simulink library "Pitch_System_Lib"  (Simulink 7.9)
settings: Solver=ode45  StartTime=0.0  StopTime=10.0  RelTol=1e-3
undefined symbols (not defined in the file or in its folder): WT_Params
libraries: mblibv1 x78, Pitch_Actuation_Lib x2, Pitch_System_Lib x1
(part 2 of 5)

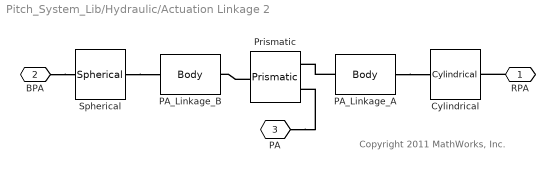
== system Pitch_System_Lib/Hydraulic/Actuation Linkage 2 ==
  note: Copyright 2011 MathWorks, Inc.
  Cylindrical : mblibv1/Joints/Cylindrical  PhysicalDomain=mechanical  SubClassName=Unknown  LeftPortType=blob  RightPortType=blob  LConnTagsString=__newl0  RConnTagsString=__newr0  UpdateFromCAD=off  NumSAPorts=0  CutJoint=off  MarkAsCut=off  Primitives=prismatic  PrimitiveProps=P1$Follower$[0 1 0]$prismatic#R1$Follower$[0 1 0]$revolute  DialogClass=JointBlock  P1Axis=[0 1 0]  R1Axis=[0 1 0]
  PA_Linkage_A : mblibv1/Bodies/Body  PhysicalDomain=mechanical  SubClassName=Unknown  LeftPortType=workingframe  RightPortType=workingframe  LConnTagsString=CS2  RConnTagsString=CS1  UpdateFromCAD=off  DialogClass=MechanicalBodyBlock  Mass=WT_Params.Pitch_Actuator.cylinder_mass  MassUnits=kg  InertiaUnits=kg*m^2  Inertia=WT_Params.Pitch_Actuator.cylinder_inertia  Shape=Cylinder  ShapeDims=[1 1]  ShapeUnits=m  ShapeUse=false  Density=1  DensityUnits=kg/m^3  DensityUse=false  GraphicsMode=MACHINE_DEFAULT  BodyColorSelMode=COLORPALETTE  BodyColor="[1     0.56863    0.011765]"  AttachedToCS=CG  CG=Left$CG$[WT_Params.Pitch_Actuator.cylinder_length/2 0 0]$CS2$CS2$m$[0 0 0]$Euler X-Y-Z$deg$CS1$false$none  WorkingFrames="Right$CS1$[WT_Params.Pitch_Actuator.cylinder_length 0 0]$CS2$CS2$m$[0 0 0]$Euler X-Y-Z$deg$Adjoining$true$none#Left$CS2$[0 0 0]$Adjoining$Adjoining$m$[0 0 0]$Euler X-Y-Z$deg$CS1$true$none#Right$CS7$[0 WT_Params.Pitch_Actuator.Geometry.outer_radius*cos(0)  WT_Params.Pitch_Actuator.Geometry.outer_radius*sin(0)]$CS1$CS1$m$[0 0 0]$Euler X-Y-Z$deg$CS1$false$none#Right$CS8$[0 WT_Params.Pitch_Actuator.Geometry.outer_radius*cos(0.2*pi)  WT_Params.Pitch_Actuator.Geometry.outer_radius*sin(0.2*pi)]$CS1$CS1$m$[0 0 0]$Euler X-Y-Z$deg$CS1$false$none#Right$CS9$[0 WT_Params.Pitch_Actuator.Geometry.outer_radius*cos(0.4*pi)  WT_Params.Pitch_Actuator.Geometry.outer_radius*sin(0.4*pi)]$CS1$CS1$m$[0 0 0]$Euler X-Y-Z$deg$CS1$false$none#Right$CS10$[0 WT_Params.Pitch_Actuator.Geometry.outer_radius*cos(0.6*pi)  WT_Params.Pitch_Actuator.Geometry.outer_radius*sin(0.6*pi)]$CS1$CS1$m$[0 0 0]$Euler X-Y-Z$deg$CS1$false$none#Right$CS11$[0 WT_Params.Pitch_Actuator.Geometry.outer_radius*cos(0.8*pi)  WT_Params.Pitch_Actuator.Geometry.outer_radius*sin(0.8*pi)]$CS1$CS1$m$[0 0 0]$Euler X-Y-Z$deg$CS1$false$none#Right$CS12$[0 WT_Params.Pitch_Actuator.Geometry.outer_radius*cos(1.0*pi)  WT_Params.Pitch_Actuator.Geometry.outer_radius*sin(1.0*pi)]$CS1$CS1$m$[0 0 0]$Euler X-Y-Z$deg$CS1$false$none#Right$CS13$[0 WT_Params.Pitch_Actuator.Geometry.outer_radius*cos(1.2*pi)  WT_Params.Pitch_Actuator.Geometry.outer_radius*sin(1.2*pi)]$CS1$CS1$m$[0 0 0]$Euler X-Y-Z$deg$CS1$false$none#Right$CS14$[0 WT_Params.Pitch_Actuator.Geometry.outer_radius*cos(1.4*pi)  WT_Params.Pitch_Actuator.Geometry.outer_radius*sin(1.4*pi)]$CS1$CS1$m$[0 0 0]$Euler X-Y-Z$deg$CS1$false$none#Right$CS15$[0 WT_Params.Pitch_Actuator.Geometry.outer_radius*cos(1.6*pi)  WT_Params.Pitch_Actuator.Geometry.outer_radius*sin(1.6*pi)]$CS1$CS1$m$[0 0 0]$Euler X-Y-Z$deg$CS1$false$none#Right$CS16$[0 WT_Params.Pitch_Actuator.Geometry.outer_radius*cos(1.8*pi)  WT_Params.Pitch_Actuator.Geometry.outer_radius*sin(1.8*pi)]$CS1$CS1$m$[0 0 0]$Euler X-Y-Z$deg$CS1$false$none#Right$CS17$[-WT_Params.Pitch_Actuator.cylinder_length WT_Params.Pitch_Actuator.Geometry.outer_radius*cos(0)  WT_Params.Pitch_Actuator.Geometry.outer_radius*sin(0)]$CS1$CS1$m$[0 0 0]$Euler X-Y-Z$deg$CS1$false$none#Right$CS18$[-WT_Params.Pitch_Actuator.cylinder_length WT_Params.Pitch_Actuator.Geometry.outer_radius*cos(0.2*pi)  WT_Params.Pitch_Actuator.Geometry.outer_radius*sin(0.2*pi)]$CS1$CS1$m$[0 0 0]$Euler X-Y-Z$deg$CS1$false$none#Right$CS19$[-WT_Params.Pitch_Actuator.cylinder_length WT_Params.Pitch_Actuator.Geometry.outer_radius*cos(0.4*pi)  WT_Params.Pitch_Actuator.Geometry.outer_radius*sin(0.4*pi)]$CS1$CS1$m$[0 0 0]$Euler X-Y-Z$deg$CS1$false$none#Right$CS20$[-WT_Params.Pitch_Actuator.cylinder_length WT_Params.Pitch_Actuator.Geometry.outer_radius*cos(0.6*pi)  WT_Params.Pitch_Actuator.Geometry.outer_radius*sin(0.6*pi)]$CS1$CS1$m$[0 0 0]$Euler X-Y-Z$deg$CS1$false$none#Right$CS21$[-WT_Params.Pitch_Actuator.cylinder_length WT_Params.Pitch_Actuator.Geometry.outer_radius*cos(0.8*pi)  WT_Params.Pitch_Actuator.Geometry.outer_radius*sin(0.8*pi)]$CS1$CS1$m$[0 0 0]$Euler X-Y-Z$deg$CS1$false$none#Right$CS22$[-WT_Params.Pitch_Actuator.cylinder_length WT_Params.Pitch_Actuator.Geometry.outer_radius*cos(1.0*pi)  WT_Params.Pitch_Actuator.Geometry.outer_radius*sin(1.0*pi)]$CS1$CS1$m$[0 0 0]$Euler X-Y-Z$deg$CS1$false$none#Right$CS23$[-WT_Params.Pitch_Actuator.cylinder_length WT_Params.Pitch_Actuator.Geometry.outer_radius*cos(1.2*pi)  WT_Params.Pitch_Actuator.Geometry.outer_radius*sin(1.2*pi)]$CS1$CS1$m$[0 0 0]$Euler X-Y-Z$deg$CS1$false$none#Right$CS24$[-WT_Params.Pitch_Actuator.cylinder_length WT_Params.Pitch_Actuator.Geometry.outer_radius*cos(1.4*pi)  WT_Params.Pitch_Actuator.Geometry.outer_radius*sin(1.4*pi)]$CS1$CS1$m$[0 0 0]$Euler X-Y-Z$deg$CS1$false$none#Right$CS25$[-WT_Params.Pitch_Actuator.cylinder_length WT_Params.Pitch_Actuator.Geometry.outer_radius*cos(1.6*pi)  WT_Params.Pitch_Actuator.Geometry.outer_radius*sin(1.6*pi)]$CS1$CS1$m$[0 0 0]$Euler X-Y-Z$deg$CS1$false$none#Right$CS26$[-WT_Params.Pitch_Actuator.cylinder_length WT_Params.Pitch_Actuator.Geometry.outer_radius*cos(1.8*pi)  WT_Params.Pitch_Actuator.Geometry.outer_radius*sin(1.8*pi)]$CS1$CS1$m$[0 0 0]$Euler X-Y-Z$deg$CS1$false$none"  CGPos=[WT_Params.Pitch_Actuator.cylinder_length/2 0 0]  CGRot=[0 0 0]  CS0Pos=[]  CS0Rot=[]  CS1Pos=[WT_Params.Pitch_Actuator.cylinder_length 0 0]  CS1Rot=[0 0 0]  CS2Pos=[0 0 0]  CS2Rot=[0 0 0]  CS3Pos=[]  CS3Rot=[]  CS4Pos=[]  CS4Rot=[]  CS5Pos=[]  CS5Rot=[]  CS6Pos=[]  CS6Rot=[]  CS7Pos="[0 WT_Params.Pitch_Actuator.Geometry.outer_radius*cos(0)  WT_Params.Pitch_Actuator.Geometry.outer_radius*sin(0)]"  CS7Rot=[0 0 0]  CS8Pos="[0 WT_Params.Pitch_Actuator.Geometry.outer_radius*cos(0.2*pi)  WT_Params.Pitch_Actuator.Geometry.outer_radius*sin(0.2*pi)]"  CS8Rot=[0 0 0]  CS9Pos="[0 WT_Params.Pitch_Actuator.Geometry.outer_radius*cos(0.4*pi)  WT_Params.Pitch_Actuator.Geometry.outer_radius*sin(0.4*pi)]"  CS9Rot=[0 0 0]  CS10Pos="[0 WT_Params.Pitch_Actuator.Geometry.outer_radius*cos(0.6*pi)  WT_Params.Pitch_Actuator.Geometry.outer_radius*sin(0.6*pi)]"  CS10Rot=[0 0 0]  CS11Pos="[0 WT_Params.Pitch_Actuator.Geometry.outer_radius*cos(0.8*pi)  WT_Params.Pitch_Actuator.Geometry.outer_radius*sin(0.8*pi)]"  CS11Rot=[0 0 0]  CS12Pos="[0 WT_Params.Pitch_Actuator.Geometry.outer_radius*cos(1.0*pi)  WT_Params.Pitch_Actuator.Geometry.outer_radius*sin(1.0*pi)]"  CS12Rot=[0 0 0]  CS13Pos="[0 WT_Params.Pitch_Actuator.Geometry.outer_radius*cos(1.2*pi)  WT_Params.Pitch_Actuator.Geometry.outer_radius*sin(1.2*pi)]"  CS13Rot=[0 0 0]  CS14Pos="[0 WT_Params.Pitch_Actuator.Geometry.outer_radius*cos(1.4*pi)  WT_Params.Pitch_Actuator.Geometry.outer_radius*sin(1.4*pi)]"  CS14Rot=[0 0 0]  CS15Pos="[0 WT_Params.Pitch_Actuator.Geometry.outer_radius*cos(1.6*pi)  WT_Params.Pitch_Actuator.Geometry.outer_radius*sin(1.6*pi)]"  CS15Rot=[0 0 0]  CS16Pos="[0 WT_Params.Pitch_Actuator.Geometry.outer_radius*cos(1.8*pi)  WT_Params.Pitch_Actuator.Geometry.outer_radius*sin(1.8*pi)]"  CS16Rot=[0 0 0]  CS17Pos="[-WT_Params.Pitch_Actuator.cylinder_length WT_Params.Pitch_Actuator.Geometry.outer_radius*cos(0)  WT_Params.Pitch_Actuator.Geometry.outer_radius*sin(0)]"  CS17Rot=[0 0 0]  CS18Pos="[-WT_Params.Pitch_Actuator.cylinder_length WT_Params.Pitch_Actuator.Geometry.outer_radius*cos(0.2*pi)  WT_Params.Pitch_Actuator.Geometry.outer_radius*sin(0.2*pi)]"  CS18Rot=[0 0 0]  CS19Pos="[-WT_Params.Pitch_Actuator.cylinder_length WT_Params.Pitch_Actuator.Geometry.outer_radius*cos(0.4*pi)  WT_Params.Pitch_Actuator.Geometry.outer_radius*sin(0.4*pi)]"  CS19Rot=[0 0 0]  CS20Pos="[-WT_Params.Pitch_Actuator.cylinder_length WT_Params.Pitch_Actuator.Geometry.outer_radius*cos(0.6*pi)  WT_Params.Pitch_Actuator.Geometry.outer_radius*sin(0.6*pi)]"  CS20Rot=[0 0 0]
  PA_Linkage_B : mblibv1/Bodies/Body  PhysicalDomain=mechanical  SubClassName=Unknown  LeftPortType=workingframe  RightPortType=workingframe  LConnTagsString=CS2  RConnTagsString=CS1  UpdateFromCAD=off  DialogClass=MechanicalBodyBlock  Mass=WT_Params.Pitch_Actuator.rod_mass  MassUnits=kg  InertiaUnits=kg*m^2  Inertia=WT_Params.Pitch_Actuator.rod_inertia  Shape=Cylinder  ShapeDims=[1 1]  ShapeUnits=m  ShapeUse=false  Density=1  DensityUnits=kg/m^3  DensityUse=false  GraphicsMode=MACHINE_DEFAULT  BodyColorSelMode=COLORPALETTE  BodyColor="[0.31373     0.31765     0.31373]"  AttachedToCS=CG  CG=Left$CG$[-WT_Params.Pitch_Actuator.cylinder_length/2 0 0]$CS1$CS1$m$[0 0 0]$Euler X-Y-Z$deg$CS1$false$none  WorkingFrames="Right$CS1$[0 0 0]$Adjoining$Adjoining$m$[0 0 0]$Euler X-Y-Z$deg$Adjoining$true$none#Left$CS2$[-WT_Params.Pitch_Actuator.cylinder_length 0 0]$CS1$CS1$m$[0 0 0]$Euler X-Y-Z$deg$CS1$true$none#Right$CS7$[0 WT_Params.Pitch_Actuator.Geometry.inner_radius*cos(0)  WT_Params.Pitch_Actuator.Geometry.inner_radius*sin(0)]$CS1$CS1$m$[0 0 0]$Euler X-Y-Z$deg$CS1$false$none#Right$CS8$[0 WT_Params.Pitch_Actuator.Geometry.inner_radius*cos(0.2*pi)  WT_Params.Pitch_Actuator.Geometry.inner_radius*sin(0.2*pi)]$CS1$CS1$m$[0 0 0]$Euler X-Y-Z$deg$CS1$false$none#Right$CS9$[0 WT_Params.Pitch_Actuator.Geometry.inner_radius*cos(0.4*pi)  WT_Params.Pitch_Actuator.Geometry.inner_radius*sin(0.4*pi)]$CS1$CS1$m$[0 0 0]$Euler X-Y-Z$deg$CS1$false$none#Right$CS10$[0 WT_Params.Pitch_Actuator.Geometry.inner_radius*cos(0.6*pi)  WT_Params.Pitch_Actuator.Geometry.inner_radius*sin(0.6*pi)]$CS1$CS1$m$[0 0 0]$Euler X-Y-Z$deg$CS1$false$none#Right$CS11$[0 WT_Params.Pitch_Actuator.Geometry.inner_radius*cos(0.8*pi)  WT_Params.Pitch_Actuator.Geometry.inner_radius*sin(0.8*pi)]$CS1$CS1$m$[0 0 0]$Euler X-Y-Z$deg$CS1$false$none#Right$CS12$[0 WT_Params.Pitch_Actuator.Geometry.inner_radius*cos(1.0*pi)  WT_Params.Pitch_Actuator.Geometry.inner_radius*sin(1.0*pi)]$CS1$CS1$m$[0 0 0]$Euler X-Y-Z$deg$CS1$false$none#Right$CS13$[0 WT_Params.Pitch_Actuator.Geometry.inner_radius*cos(1.2*pi)  WT_Params.Pitch_Actuator.Geometry.inner_radius*sin(1.2*pi)]$CS1$CS1$m$[0 0 0]$Euler X-Y-Z$deg$CS1$false$none#Right$CS14$[0 WT_Params.Pitch_Actuator.Geometry.inner_radius*cos(1.4*pi)  WT_Params.Pitch_Actuator.Geometry.inner_radius*sin(1.4*pi)]$CS1$CS1$m$[0 0 0]$Euler X-Y-Z$deg$CS1$false$none#Right$CS15$[0 WT_Params.Pitch_Actuator.Geometry.inner_radius*cos(1.6*pi)  WT_Params.Pitch_Actuator.Geometry.inner_radius*sin(1.6*pi)]$CS1$CS1$m$[0 0 0]$Euler X-Y-Z$deg$CS1$false$none#Right$CS16$[0 WT_Params.Pitch_Actuator.Geometry.inner_radius*cos(1.8*pi)  WT_Params.Pitch_Actuator.Geometry.inner_radius*sin(1.8*pi)]$CS1$CS1$m$[0 0 0]$Euler X-Y-Z$deg$CS1$false$none#Right$CS17$[-WT_Params.Pitch_Actuator.cylinder_length WT_Params.Pitch_Actuator.Geometry.inner_radius*cos(0)  WT_Params.Pitch_Actuator.Geometry.inner_radius*sin(0)]$CS1$CS1$m$[0 0 0]$Euler X-Y-Z$deg$CS1$false$none#Right$CS18$[-WT_Params.Pitch_Actuator.cylinder_length WT_Params.Pitch_Actuator.Geometry.inner_radius*cos(0.2*pi)  WT_Params.Pitch_Actuator.Geometry.inner_radius*sin(0.2*pi)]$CS1$CS1$m$[0 0 0]$Euler X-Y-Z$deg$CS1$false$none#Right$CS19$[-WT_Params.Pitch_Actuator.cylinder_length WT_Params.Pitch_Actuator.Geometry.inner_radius*cos(0.4*pi)  WT_Params.Pitch_Actuator.Geometry.inner_radius*sin(0.4*pi)]$CS1$CS1$m$[0 0 0]$Euler X-Y-Z$deg$CS1$false$none#Right$CS20$[-WT_Params.Pitch_Actuator.cylinder_length WT_Params.Pitch_Actuator.Geometry.inner_radius*cos(0.6*pi)  WT_Params.Pitch_Actuator.Geometry.inner_radius*sin(0.6*pi)]$CS1$CS1$m$[0 0 0]$Euler X-Y-Z$deg$CS1$false$none#Right$CS21$[-WT_Params.Pitch_Actuator.cylinder_length WT_Params.Pitch_Actuator.Geometry.inner_radius*cos(0.8*pi)  WT_Params.Pitch_Actuator.Geometry.inner_radius*sin(0.8*pi)]$CS1$CS1$m$[0 0 0]$Euler X-Y-Z$deg$CS1$false$none#Right$CS22$[-WT_Params.Pitch_Actuator.cylinder_length WT_Params.Pitch_Actuator.Geometry.inner_radius*cos(1.0*pi)  WT_Params.Pitch_Actuator.Geometry.inner_radius*sin(1.0*pi)]$CS1$CS1$m$[0 0 0]$Euler X-Y-Z$deg$CS1$false$none#Right$CS23$[-WT_Params.Pitch_Actuator.cylinder_length WT_Params.Pitch_Actuator.Geometry.inner_radius*cos(1.2*pi)  WT_Params.Pitch_Actuator.Geometry.inner_radius*sin(1.2*pi)]$CS1$CS1$m$[0 0 0]$Euler X-Y-Z$deg$CS1$false$none#Right$CS24$[-WT_Params.Pitch_Actuator.cylinder_length WT_Params.Pitch_Actuator.Geometry.inner_radius*cos(1.4*pi)  WT_Params.Pitch_Actuator.Geometry.inner_radius*sin(1.4*pi)]$CS1$CS1$m$[0 0 0]$Euler X-Y-Z$deg$CS1$false$none#Right$CS25$[-WT_Params.Pitch_Actuator.cylinder_length WT_Params.Pitch_Actuator.Geometry.inner_radius*cos(1.6*pi)  WT_Params.Pitch_Actuator.Geometry.inner_radius*sin(1.6*pi)]$CS1$CS1$m$[0 0 0]$Euler X-Y-Z$deg$CS1$false$none#Right$CS26$[-WT_Params.Pitch_Actuator.cylinder_length WT_Params.Pitch_Actuator.Geometry.inner_radius*cos(1.8*pi)  WT_Params.Pitch_Actuator.Geometry.inner_radius*sin(1.8*pi)]$CS1$CS1$m$[0 0 0]$Euler X-Y-Z$deg$CS1$false$none"  CGPos=[-WT_Params.Pitch_Actuator.cylinder_length/2 0 0]  CGRot=[0 0 0]  CS0Pos=[]  CS0Rot=[]  CS1Pos=[0 0 0]  CS1Rot=[0 0 0]  CS2Pos=[-WT_Params.Pitch_Actuator.cylinder_length 0 0]  CS2Rot=[0 0 0]  CS3Pos=[]  CS3Rot=[]  CS4Pos=[]  CS4Rot=[]  CS5Pos=[]  CS5Rot=[]  CS6Pos=[]  CS6Rot=[]  CS7Pos="[0 WT_Params.Pitch_Actuator.Geometry.inner_radius*cos(0)  WT_Params.Pitch_Actuator.Geometry.inner_radius*sin(0)]"  CS7Rot=[0 0 0]  CS8Pos="[0 WT_Params.Pitch_Actuator.Geometry.inner_radius*cos(0.2*pi)  WT_Params.Pitch_Actuator.Geometry.inner_radius*sin(0.2*pi)]"  CS8Rot=[0 0 0]  CS9Pos="[0 WT_Params.Pitch_Actuator.Geometry.inner_radius*cos(0.4*pi)  WT_Params.Pitch_Actuator.Geometry.inner_radius*sin(0.4*pi)]"  CS9Rot=[0 0 0]  CS10Pos="[0 WT_Params.Pitch_Actuator.Geometry.inner_radius*cos(0.6*pi)  WT_Params.Pitch_Actuator.Geometry.inner_radius*sin(0.6*pi)]"  CS10Rot=[0 0 0]  CS11Pos="[0 WT_Params.Pitch_Actuator.Geometry.inner_radius*cos(0.8*pi)  WT_Params.Pitch_Actuator.Geometry.inner_radius*sin(0.8*pi)]"  CS11Rot=[0 0 0]  CS12Pos="[0 WT_Params.Pitch_Actuator.Geometry.inner_radius*cos(1.0*pi)  WT_Params.Pitch_Actuator.Geometry.inner_radius*sin(1.0*pi)]"  CS12Rot=[0 0 0]  CS13Pos="[0 WT_Params.Pitch_Actuator.Geometry.inner_radius*cos(1.2*pi)  WT_Params.Pitch_Actuator.Geometry.inner_radius*sin(1.2*pi)]"  CS13Rot=[0 0 0]  CS14Pos="[0 WT_Params.Pitch_Actuator.Geometry.inner_radius*cos(1.4*pi)  WT_Params.Pitch_Actuator.Geometry.inner_radius*sin(1.4*pi)]"  CS14Rot=[0 0 0]  CS15Pos="[0 WT_Params.Pitch_Actuator.Geometry.inner_radius*cos(1.6*pi)  WT_Params.Pitch_Actuator.Geometry.inner_radius*sin(1.6*pi)]"  CS15Rot=[0 0 0]  CS16Pos="[0 WT_Params.Pitch_Actuator.Geometry.inner_radius*cos(1.8*pi)  WT_Params.Pitch_Actuator.Geometry.inner_radius*sin(1.8*pi)]"  CS16Rot=[0 0 0]  CS17Pos="[-WT_Params.Pitch_Actuator.cylinder_length WT_Params.Pitch_Actuator.Geometry.inner_radius*cos(0)  WT_Params.Pitch_Actuator.Geometry.inner_radius*sin(0)]"  CS17Rot=[0 0 0]  CS18Pos="[-WT_Params.Pitch_Actuator.cylinder_length WT_Params.Pitch_Actuator.Geometry.inner_radius*cos(0.2*pi)  WT_Params.Pitch_Actuator.Geometry.inner_radius*sin(0.2*pi)]"  CS18Rot=[0 0 0]  CS19Pos="[-WT_Params.Pitch_Actuator.cylinder_length WT_Params.Pitch_Actuator.Geometry.inner_radius*cos(0.4*pi)  WT_Params.Pitch_Actuator.Geometry.inner_radius*sin(0.4*pi)]"  CS19Rot=[0 0 0]  CS20Pos="[-WT_Params.Pitch_Actuator.cylinder_length WT_Params.Pitch_Actuator.Geometry.inner_radius*cos(0.6*pi)  WT_Params.Pitch_Actuator.Geometry.inner_radius*sin(0.6*pi)]"  CS20Rot=[0 0 0]
  Prismatic : mblibv1/Joints/Prismatic  PhysicalDomain=mechanical  SubClassName=Unknown  LeftPortType=blob  RightPortType=blob  LConnTagsString=__newl0|SA1  RConnTagsString=__newr0  UpdateFromCAD=off  NumSAPorts=1  CutJoint=off  MarkAsCut=off  Primitives=prismatic  PrimitiveProps=P1$Base$[1 0 0]$prismatic  DialogClass=JointBlock  P1Axis=[1 0 0]
  Spherical : mblibv1/Joints/Spherical  LConnTagsString=__newl0  RConnTagsString=__newr0  UpdateFromCAD=off  NumSAPorts=0  CutJoint=off  MarkAsCut=off  Primitives=spherical  PrimitiveProps=S$WORLD$[0 0 0]$spherical  DialogClass=JointBlock  SAxis=[0 0 0]
  RPA : PMIOPort  Port=1  Side=Right
  BPA : PMIOPort  Port=2  Side=Left
  PA : PMIOPort  Tag=PMCPort  Port=3  Side=Left
  connections:
  PA_Linkage_A/RConn1 -- Prismatic/LConn1
  PA_Linkage_A/LConn1 -- Cylindrical/LConn1
  Spherical/RConn1 -- PA_Linkage_B/RConn1
  Prismatic/RConn1 -- PA_Linkage_B/LConn1
  PA/RConn1 -- Prismatic/LConn2
  RPA/RConn1 -- Cylindrical/RConn1
  BPA/RConn1 -- Spherical/LConn1

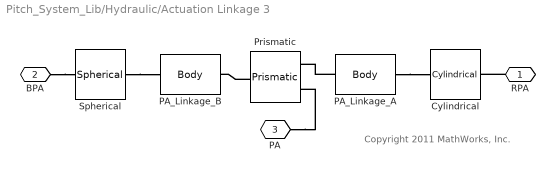
== system Pitch_System_Lib/Hydraulic/Actuation Linkage 3 ==
  note: Copyright 2011 MathWorks, Inc.
  Cylindrical : mblibv1/Joints/Cylindrical  PhysicalDomain=mechanical  SubClassName=Unknown  LeftPortType=blob  RightPortType=blob  LConnTagsString=__newl0  RConnTagsString=__newr0  UpdateFromCAD=off  NumSAPorts=0  CutJoint=off  MarkAsCut=off  Primitives=prismatic  PrimitiveProps=P1$Follower$[0 1 0]$prismatic#R1$Follower$[0 1 0]$revolute  DialogClass=JointBlock  P1Axis=[0 1 0]  R1Axis=[0 1 0]
  PA_Linkage_A : mblibv1/Bodies/Body  PhysicalDomain=mechanical  SubClassName=Unknown  LeftPortType=workingframe  RightPortType=workingframe  LConnTagsString=CS2  RConnTagsString=CS1  UpdateFromCAD=off  DialogClass=MechanicalBodyBlock  Mass=WT_Params.Pitch_Actuator.cylinder_mass  MassUnits=kg  InertiaUnits=kg*m^2  Inertia=WT_Params.Pitch_Actuator.cylinder_inertia  Shape=Cylinder  ShapeDims=[1 1]  ShapeUnits=m  ShapeUse=false  Density=1  DensityUnits=kg/m^3  DensityUse=false  GraphicsMode=MACHINE_DEFAULT  BodyColorSelMode=COLORPALETTE  BodyColor="[1     0.56863    0.011765]"  AttachedToCS=CG  CG=Left$CG$[WT_Params.Pitch_Actuator.cylinder_length/2 0 0]$CS2$CS2$m$[0 0 0]$Euler X-Y-Z$deg$CS1$false$none  WorkingFrames="Right$CS1$[WT_Params.Pitch_Actuator.cylinder_length 0 0]$CS2$CS2$m$[0 0 0]$Euler X-Y-Z$deg$Adjoining$true$none#Left$CS2$[0 0 0]$Adjoining$Adjoining$m$[0 0 0]$Euler X-Y-Z$deg$CS1$true$none#Right$CS7$[0 WT_Params.Pitch_Actuator.Geometry.outer_radius*cos(0)  WT_Params.Pitch_Actuator.Geometry.outer_radius*sin(0)]$CS1$CS1$m$[0 0 0]$Euler X-Y-Z$deg$CS1$false$none#Right$CS8$[0 WT_Params.Pitch_Actuator.Geometry.outer_radius*cos(0.2*pi)  WT_Params.Pitch_Actuator.Geometry.outer_radius*sin(0.2*pi)]$CS1$CS1$m$[0 0 0]$Euler X-Y-Z$deg$CS1$false$none#Right$CS9$[0 WT_Params.Pitch_Actuator.Geometry.outer_radius*cos(0.4*pi)  WT_Params.Pitch_Actuator.Geometry.outer_radius*sin(0.4*pi)]$CS1$CS1$m$[0 0 0]$Euler X-Y-Z$deg$CS1$false$none#Right$CS10$[0 WT_Params.Pitch_Actuator.Geometry.outer_radius*cos(0.6*pi)  WT_Params.Pitch_Actuator.Geometry.outer_radius*sin(0.6*pi)]$CS1$CS1$m$[0 0 0]$Euler X-Y-Z$deg$CS1$false$none#Right$CS11$[0 WT_Params.Pitch_Actuator.Geometry.outer_radius*cos(0.8*pi)  WT_Params.Pitch_Actuator.Geometry.outer_radius*sin(0.8*pi)]$CS1$CS1$m$[0 0 0]$Euler X-Y-Z$deg$CS1$false$none#Right$CS12$[0 WT_Params.Pitch_Actuator.Geometry.outer_radius*cos(1.0*pi)  WT_Params.Pitch_Actuator.Geometry.outer_radius*sin(1.0*pi)]$CS1$CS1$m$[0 0 0]$Euler X-Y-Z$deg$CS1$false$none#Right$CS13$[0 WT_Params.Pitch_Actuator.Geometry.outer_radius*cos(1.2*pi)  WT_Params.Pitch_Actuator.Geometry.outer_radius*sin(1.2*pi)]$CS1$CS1$m$[0 0 0]$Euler X-Y-Z$deg$CS1$false$none#Right$CS14$[0 WT_Params.Pitch_Actuator.Geometry.outer_radius*cos(1.4*pi)  WT_Params.Pitch_Actuator.Geometry.outer_radius*sin(1.4*pi)]$CS1$CS1$m$[0 0 0]$Euler X-Y-Z$deg$CS1$false$none#Right$CS15$[0 WT_Params.Pitch_Actuator.Geometry.outer_radius*cos(1.6*pi)  WT_Params.Pitch_Actuator.Geometry.outer_radius*sin(1.6*pi)]$CS1$CS1$m$[0 0 0]$Euler X-Y-Z$deg$CS1$false$none#Right$CS16$[0 WT_Params.Pitch_Actuator.Geometry.outer_radius*cos(1.8*pi)  WT_Params.Pitch_Actuator.Geometry.outer_radius*sin(1.8*pi)]$CS1$CS1$m$[0 0 0]$Euler X-Y-Z$deg$CS1$false$none#Right$CS17$[-WT_Params.Pitch_Actuator.cylinder_length WT_Params.Pitch_Actuator.Geometry.outer_radius*cos(0)  WT_Params.Pitch_Actuator.Geometry.outer_radius*sin(0)]$CS1$CS1$m$[0 0 0]$Euler X-Y-Z$deg$CS1$false$none#Right$CS18$[-WT_Params.Pitch_Actuator.cylinder_length WT_Params.Pitch_Actuator.Geometry.outer_radius*cos(0.2*pi)  WT_Params.Pitch_Actuator.Geometry.outer_radius*sin(0.2*pi)]$CS1$CS1$m$[0 0 0]$Euler X-Y-Z$deg$CS1$false$none#Right$CS19$[-WT_Params.Pitch_Actuator.cylinder_length WT_Params.Pitch_Actuator.Geometry.outer_radius*cos(0.4*pi)  WT_Params.Pitch_Actuator.Geometry.outer_radius*sin(0.4*pi)]$CS1$CS1$m$[0 0 0]$Euler X-Y-Z$deg$CS1$false$none#Right$CS20$[-WT_Params.Pitch_Actuator.cylinder_length WT_Params.Pitch_Actuator.Geometry.outer_radius*cos(0.6*pi)  WT_Params.Pitch_Actuator.Geometry.outer_radius*sin(0.6*pi)]$CS1$CS1$m$[0 0 0]$Euler X-Y-Z$deg$CS1$false$none#Right$CS21$[-WT_Params.Pitch_Actuator.cylinder_length WT_Params.Pitch_Actuator.Geometry.outer_radius*cos(0.8*pi)  WT_Params.Pitch_Actuator.Geometry.outer_radius*sin(0.8*pi)]$CS1$CS1$m$[0 0 0]$Euler X-Y-Z$deg$CS1$false$none#Right$CS22$[-WT_Params.Pitch_Actuator.cylinder_length WT_Params.Pitch_Actuator.Geometry.outer_radius*cos(1.0*pi)  WT_Params.Pitch_Actuator.Geometry.outer_radius*sin(1.0*pi)]$CS1$CS1$m$[0 0 0]$Euler X-Y-Z$deg$CS1$false$none#Right$CS23$[-WT_Params.Pitch_Actuator.cylinder_length WT_Params.Pitch_Actuator.Geometry.outer_radius*cos(1.2*pi)  WT_Params.Pitch_Actuator.Geometry.outer_radius*sin(1.2*pi)]$CS1$CS1$m$[0 0 0]$Euler X-Y-Z$deg$CS1$false$none#Right$CS24$[-WT_Params.Pitch_Actuator.cylinder_length WT_Params.Pitch_Actuator.Geometry.outer_radius*cos(1.4*pi)  WT_Params.Pitch_Actuator.Geometry.outer_radius*sin(1.4*pi)]$CS1$CS1$m$[0 0 0]$Euler X-Y-Z$deg$CS1$false$none#Right$CS25$[-WT_Params.Pitch_Actuator.cylinder_length WT_Params.Pitch_Actuator.Geometry.outer_radius*cos(1.6*pi)  WT_Params.Pitch_Actuator.Geometry.outer_radius*sin(1.6*pi)]$CS1$CS1$m$[0 0 0]$Euler X-Y-Z$deg$CS1$false$none#Right$CS26$[-WT_Params.Pitch_Actuator.cylinder_length WT_Params.Pitch_Actuator.Geometry.outer_radius*cos(1.8*pi)  WT_Params.Pitch_Actuator.Geometry.outer_radius*sin(1.8*pi)]$CS1$CS1$m$[0 0 0]$Euler X-Y-Z$deg$CS1$false$none"  CGPos=[WT_Params.Pitch_Actuator.cylinder_length/2 0 0]  CGRot=[0 0 0]  CS0Pos=[]  CS0Rot=[]  CS1Pos=[WT_Params.Pitch_Actuator.cylinder_length 0 0]  CS1Rot=[0 0 0]  CS2Pos=[0 0 0]  CS2Rot=[0 0 0]  CS3Pos=[]  CS3Rot=[]  CS4Pos=[]  CS4Rot=[]  CS5Pos=[]  CS5Rot=[]  CS6Pos=[]  CS6Rot=[]  CS7Pos="[0 WT_Params.Pitch_Actuator.Geometry.outer_radius*cos(0)  WT_Params.Pitch_Actuator.Geometry.outer_radius*sin(0)]"  CS7Rot=[0 0 0]  CS8Pos="[0 WT_Params.Pitch_Actuator.Geometry.outer_radius*cos(0.2*pi)  WT_Params.Pitch_Actuator.Geometry.outer_radius*sin(0.2*pi)]"  CS8Rot=[0 0 0]  CS9Pos="[0 WT_Params.Pitch_Actuator.Geometry.outer_radius*cos(0.4*pi)  WT_Params.Pitch_Actuator.Geometry.outer_radius*sin(0.4*pi)]"  CS9Rot=[0 0 0]  CS10Pos="[0 WT_Params.Pitch_Actuator.Geometry.outer_radius*cos(0.6*pi)  WT_Params.Pitch_Actuator.Geometry.outer_radius*sin(0.6*pi)]"  CS10Rot=[0 0 0]  CS11Pos="[0 WT_Params.Pitch_Actuator.Geometry.outer_radius*cos(0.8*pi)  WT_Params.Pitch_Actuator.Geometry.outer_radius*sin(0.8*pi)]"  CS11Rot=[0 0 0]  CS12Pos="[0 WT_Params.Pitch_Actuator.Geometry.outer_radius*cos(1.0*pi)  WT_Params.Pitch_Actuator.Geometry.outer_radius*sin(1.0*pi)]"  CS12Rot=[0 0 0]  CS13Pos="[0 WT_Params.Pitch_Actuator.Geometry.outer_radius*cos(1.2*pi)  WT_Params.Pitch_Actuator.Geometry.outer_radius*sin(1.2*pi)]"  CS13Rot=[0 0 0]  CS14Pos="[0 WT_Params.Pitch_Actuator.Geometry.outer_radius*cos(1.4*pi)  WT_Params.Pitch_Actuator.Geometry.outer_radius*sin(1.4*pi)]"  CS14Rot=[0 0 0]  CS15Pos="[0 WT_Params.Pitch_Actuator.Geometry.outer_radius*cos(1.6*pi)  WT_Params.Pitch_Actuator.Geometry.outer_radius*sin(1.6*pi)]"  CS15Rot=[0 0 0]  CS16Pos="[0 WT_Params.Pitch_Actuator.Geometry.outer_radius*cos(1.8*pi)  WT_Params.Pitch_Actuator.Geometry.outer_radius*sin(1.8*pi)]"  CS16Rot=[0 0 0]  CS17Pos="[-WT_Params.Pitch_Actuator.cylinder_length WT_Params.Pitch_Actuator.Geometry.outer_radius*cos(0)  WT_Params.Pitch_Actuator.Geometry.outer_radius*sin(0)]"  CS17Rot=[0 0 0]  CS18Pos="[-WT_Params.Pitch_Actuator.cylinder_length WT_Params.Pitch_Actuator.Geometry.outer_radius*cos(0.2*pi)  WT_Params.Pitch_Actuator.Geometry.outer_radius*sin(0.2*pi)]"  CS18Rot=[0 0 0]  CS19Pos="[-WT_Params.Pitch_Actuator.cylinder_length WT_Params.Pitch_Actuator.Geometry.outer_radius*cos(0.4*pi)  WT_Params.Pitch_Actuator.Geometry.outer_radius*sin(0.4*pi)]"  CS19Rot=[0 0 0]  CS20Pos="[-WT_Params.Pitch_Actuator.cylinder_length WT_Params.Pitch_Actuator.Geometry.outer_radius*cos(0.6*pi)  WT_Params.Pitch_Actuator.Geometry.outer_radius*sin(0.6*pi)]"  CS20Rot=[0 0 0]
  PA_Linkage_B : mblibv1/Bodies/Body  PhysicalDomain=mechanical  SubClassName=Unknown  LeftPortType=workingframe  RightPortType=workingframe  LConnTagsString=CS2  RConnTagsString=CS1  UpdateFromCAD=off  DialogClass=MechanicalBodyBlock  Mass=WT_Params.Pitch_Actuator.rod_mass  MassUnits=kg  InertiaUnits=kg*m^2  Inertia=WT_Params.Pitch_Actuator.rod_inertia  Shape=Cylinder  ShapeDims=[1 1]  ShapeUnits=m  ShapeUse=false  Density=1  DensityUnits=kg/m^3  DensityUse=false  GraphicsMode=MACHINE_DEFAULT  BodyColorSelMode=COLORPALETTE  BodyColor="[0.31373     0.31765     0.31373]"  AttachedToCS=CG  CG=Left$CG$[-WT_Params.Pitch_Actuator.cylinder_length/2 0 0]$CS1$CS1$m$[0 0 0]$Euler X-Y-Z$deg$CS1$false$none  WorkingFrames="Right$CS1$[0 0 0]$Adjoining$Adjoining$m$[0 0 0]$Euler X-Y-Z$deg$Adjoining$true$none#Left$CS2$[-WT_Params.Pitch_Actuator.cylinder_length 0 0]$CS1$CS1$m$[0 0 0]$Euler X-Y-Z$deg$CS1$true$none#Right$CS7$[0 WT_Params.Pitch_Actuator.Geometry.inner_radius*cos(0)  WT_Params.Pitch_Actuator.Geometry.inner_radius*sin(0)]$CS1$CS1$m$[0 0 0]$Euler X-Y-Z$deg$CS1$false$none#Right$CS8$[0 WT_Params.Pitch_Actuator.Geometry.inner_radius*cos(0.2*pi)  WT_Params.Pitch_Actuator.Geometry.inner_radius*sin(0.2*pi)]$CS1$CS1$m$[0 0 0]$Euler X-Y-Z$deg$CS1$false$none#Right$CS9$[0 WT_Params.Pitch_Actuator.Geometry.inner_radius*cos(0.4*pi)  WT_Params.Pitch_Actuator.Geometry.inner_radius*sin(0.4*pi)]$CS1$CS1$m$[0 0 0]$Euler X-Y-Z$deg$CS1$false$none#Right$CS10$[0 WT_Params.Pitch_Actuator.Geometry.inner_radius*cos(0.6*pi)  WT_Params.Pitch_Actuator.Geometry.inner_radius*sin(0.6*pi)]$CS1$CS1$m$[0 0 0]$Euler X-Y-Z$deg$CS1$false$none#Right$CS11$[0 WT_Params.Pitch_Actuator.Geometry.inner_radius*cos(0.8*pi)  WT_Params.Pitch_Actuator.Geometry.inner_radius*sin(0.8*pi)]$CS1$CS1$m$[0 0 0]$Euler X-Y-Z$deg$CS1$false$none#Right$CS12$[0 WT_Params.Pitch_Actuator.Geometry.inner_radius*cos(1.0*pi)  WT_Params.Pitch_Actuator.Geometry.inner_radius*sin(1.0*pi)]$CS1$CS1$m$[0 0 0]$Euler X-Y-Z$deg$CS1$false$none#Right$CS13$[0 WT_Params.Pitch_Actuator.Geometry.inner_radius*cos(1.2*pi)  WT_Params.Pitch_Actuator.Geometry.inner_radius*sin(1.2*pi)]$CS1$CS1$m$[0 0 0]$Euler X-Y-Z$deg$CS1$false$none#Right$CS14$[0 WT_Params.Pitch_Actuator.Geometry.inner_radius*cos(1.4*pi)  WT_Params.Pitch_Actuator.Geometry.inner_radius*sin(1.4*pi)]$CS1$CS1$m$[0 0 0]$Euler X-Y-Z$deg$CS1$false$none#Right$CS15$[0 WT_Params.Pitch_Actuator.Geometry.inner_radius*cos(1.6*pi)  WT_Params.Pitch_Actuator.Geometry.inner_radius*sin(1.6*pi)]$CS1$CS1$m$[0 0 0]$Euler X-Y-Z$deg$CS1$false$none#Right$CS16$[0 WT_Params.Pitch_Actuator.Geometry.inner_radius*cos(1.8*pi)  WT_Params.Pitch_Actuator.Geometry.inner_radius*sin(1.8*pi)]$CS1$CS1$m$[0 0 0]$Euler X-Y-Z$deg$CS1$false$none#Right$CS17$[-WT_Params.Pitch_Actuator.cylinder_length WT_Params.Pitch_Actuator.Geometry.inner_radius*cos(0)  WT_Params.Pitch_Actuator.Geometry.inner_radius*sin(0)]$CS1$CS1$m$[0 0 0]$Euler X-Y-Z$deg$CS1$false$none#Right$CS18$[-WT_Params.Pitch_Actuator.cylinder_length WT_Params.Pitch_Actuator.Geometry.inner_radius*cos(0.2*pi)  WT_Params.Pitch_Actuator.Geometry.inner_radius*sin(0.2*pi)]$CS1$CS1$m$[0 0 0]$Euler X-Y-Z$deg$CS1$false$none#Right$CS19$[-WT_Params.Pitch_Actuator.cylinder_length WT_Params.Pitch_Actuator.Geometry.inner_radius*cos(0.4*pi)  WT_Params.Pitch_Actuator.Geometry.inner_radius*sin(0.4*pi)]$CS1$CS1$m$[0 0 0]$Euler X-Y-Z$deg$CS1$false$none#Right$CS20$[-WT_Params.Pitch_Actuator.cylinder_length WT_Params.Pitch_Actuator.Geometry.inner_radius*cos(0.6*pi)  WT_Params.Pitch_Actuator.Geometry.inner_radius*sin(0.6*pi)]$CS1$CS1$m$[0 0 0]$Euler X-Y-Z$deg$CS1$false$none#Right$CS21$[-WT_Params.Pitch_Actuator.cylinder_length WT_Params.Pitch_Actuator.Geometry.inner_radius*cos(0.8*pi)  WT_Params.Pitch_Actuator.Geometry.inner_radius*sin(0.8*pi)]$CS1$CS1$m$[0 0 0]$Euler X-Y-Z$deg$CS1$false$none#Right$CS22$[-WT_Params.Pitch_Actuator.cylinder_length WT_Params.Pitch_Actuator.Geometry.inner_radius*cos(1.0*pi)  WT_Params.Pitch_Actuator.Geometry.inner_radius*sin(1.0*pi)]$CS1$CS1$m$[0 0 0]$Euler X-Y-Z$deg$CS1$false$none#Right$CS23$[-WT_Params.Pitch_Actuator.cylinder_length WT_Params.Pitch_Actuator.Geometry.inner_radius*cos(1.2*pi)  WT_Params.Pitch_Actuator.Geometry.inner_radius*sin(1.2*pi)]$CS1$CS1$m$[0 0 0]$Euler X-Y-Z$deg$CS1$false$none#Right$CS24$[-WT_Params.Pitch_Actuator.cylinder_length WT_Params.Pitch_Actuator.Geometry.inner_radius*cos(1.4*pi)  WT_Params.Pitch_Actuator.Geometry.inner_radius*sin(1.4*pi)]$CS1$CS1$m$[0 0 0]$Euler X-Y-Z$deg$CS1$false$none#Right$CS25$[-WT_Params.Pitch_Actuator.cylinder_length WT_Params.Pitch_Actuator.Geometry.inner_radius*cos(1.6*pi)  WT_Params.Pitch_Actuator.Geometry.inner_radius*sin(1.6*pi)]$CS1$CS1$m$[0 0 0]$Euler X-Y-Z$deg$CS1$false$none#Right$CS26$[-WT_Params.Pitch_Actuator.cylinder_length WT_Params.Pitch_Actuator.Geometry.inner_radius*cos(1.8*pi)  WT_Params.Pitch_Actuator.Geometry.inner_radius*sin(1.8*pi)]$CS1$CS1$m$[0 0 0]$Euler X-Y-Z$deg$CS1$false$none"  CGPos=[-WT_Params.Pitch_Actuator.cylinder_length/2 0 0]  CGRot=[0 0 0]  CS0Pos=[]  CS0Rot=[]  CS1Pos=[0 0 0]  CS1Rot=[0 0 0]  CS2Pos=[-WT_Params.Pitch_Actuator.cylinder_length 0 0]  CS2Rot=[0 0 0]  CS3Pos=[]  CS3Rot=[]  CS4Pos=[]  CS4Rot=[]  CS5Pos=[]  CS5Rot=[]  CS6Pos=[]  CS6Rot=[]  CS7Pos="[0 WT_Params.Pitch_Actuator.Geometry.inner_radius*cos(0)  WT_Params.Pitch_Actuator.Geometry.inner_radius*sin(0)]"  CS7Rot=[0 0 0]  CS8Pos="[0 WT_Params.Pitch_Actuator.Geometry.inner_radius*cos(0.2*pi)  WT_Params.Pitch_Actuator.Geometry.inner_radius*sin(0.2*pi)]"  CS8Rot=[0 0 0]  CS9Pos="[0 WT_Params.Pitch_Actuator.Geometry.inner_radius*cos(0.4*pi)  WT_Params.Pitch_Actuator.Geometry.inner_radius*sin(0.4*pi)]"  CS9Rot=[0 0 0]  CS10Pos="[0 WT_Params.Pitch_Actuator.Geometry.inner_radius*cos(0.6*pi)  WT_Params.Pitch_Actuator.Geometry.inner_radius*sin(0.6*pi)]"  CS10Rot=[0 0 0]  CS11Pos="[0 WT_Params.Pitch_Actuator.Geometry.inner_radius*cos(0.8*pi)  WT_Params.Pitch_Actuator.Geometry.inner_radius*sin(0.8*pi)]"  CS11Rot=[0 0 0]  CS12Pos="[0 WT_Params.Pitch_Actuator.Geometry.inner_radius*cos(1.0*pi)  WT_Params.Pitch_Actuator.Geometry.inner_radius*sin(1.0*pi)]"  CS12Rot=[0 0 0]  CS13Pos="[0 WT_Params.Pitch_Actuator.Geometry.inner_radius*cos(1.2*pi)  WT_Params.Pitch_Actuator.Geometry.inner_radius*sin(1.2*pi)]"  CS13Rot=[0 0 0]  CS14Pos="[0 WT_Params.Pitch_Actuator.Geometry.inner_radius*cos(1.4*pi)  WT_Params.Pitch_Actuator.Geometry.inner_radius*sin(1.4*pi)]"  CS14Rot=[0 0 0]  CS15Pos="[0 WT_Params.Pitch_Actuator.Geometry.inner_radius*cos(1.6*pi)  WT_Params.Pitch_Actuator.Geometry.inner_radius*sin(1.6*pi)]"  CS15Rot=[0 0 0]  CS16Pos="[0 WT_Params.Pitch_Actuator.Geometry.inner_radius*cos(1.8*pi)  WT_Params.Pitch_Actuator.Geometry.inner_radius*sin(1.8*pi)]"  CS16Rot=[0 0 0]  CS17Pos="[-WT_Params.Pitch_Actuator.cylinder_length WT_Params.Pitch_Actuator.Geometry.inner_radius*cos(0)  WT_Params.Pitch_Actuator.Geometry.inner_radius*sin(0)]"  CS17Rot=[0 0 0]  CS18Pos="[-WT_Params.Pitch_Actuator.cylinder_length WT_Params.Pitch_Actuator.Geometry.inner_radius*cos(0.2*pi)  WT_Params.Pitch_Actuator.Geometry.inner_radius*sin(0.2*pi)]"  CS18Rot=[0 0 0]  CS19Pos="[-WT_Params.Pitch_Actuator.cylinder_length WT_Params.Pitch_Actuator.Geometry.inner_radius*cos(0.4*pi)  WT_Params.Pitch_Actuator.Geometry.inner_radius*sin(0.4*pi)]"  CS19Rot=[0 0 0]  CS20Pos="[-WT_Params.Pitch_Actuator.cylinder_length WT_Params.Pitch_Actuator.Geometry.inner_radius*cos(0.6*pi)  WT_Params.Pitch_Actuator.Geometry.inner_radius*sin(0.6*pi)]"  CS20Rot=[0 0 0]
  Prismatic : mblibv1/Joints/Prismatic  PhysicalDomain=mechanical  SubClassName=Unknown  LeftPortType=blob  RightPortType=blob  LConnTagsString=__newl0|SA1  RConnTagsString=__newr0  UpdateFromCAD=off  NumSAPorts=1  CutJoint=off  MarkAsCut=off  Primitives=prismatic  PrimitiveProps=P1$Base$[1 0 0]$prismatic  DialogClass=JointBlock  P1Axis=[1 0 0]
  Spherical : mblibv1/Joints/Spherical  LConnTagsString=__newl0  RConnTagsString=__newr0  UpdateFromCAD=off  NumSAPorts=0  CutJoint=off  MarkAsCut=off  Primitives=spherical  PrimitiveProps=S$WORLD$[0 0 0]$spherical  DialogClass=JointBlock  SAxis=[0 0 0]
  RPA : PMIOPort  Port=1  Side=Right
  BPA : PMIOPort  Port=2  Side=Left
  PA : PMIOPort  Tag=PMCPort  Port=3  Side=Left
  connections:
  BPA/RConn1 -- Spherical/LConn1
  RPA/RConn1 -- Cylindrical/RConn1
  PA/RConn1 -- Prismatic/LConn2
  Prismatic/RConn1 -- PA_Linkage_B/LConn1
  Spherical/RConn1 -- PA_Linkage_B/RConn1
  PA_Linkage_A/LConn1 -- Cylindrical/LConn1
  PA_Linkage_A/RConn1 -- Prismatic/LConn1

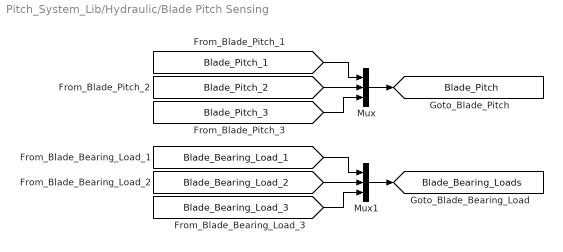
== system Pitch_System_Lib/Hydraulic/Blade Pitch Sensing ==
  Mux : Mux  Inputs=3
  Mux1 : Mux  Inputs=3
  tag scope: Blade_Bearing_Loads=global, Blade_Pitch=global
  wires:
  Mux1/1 -> [Blade_Bearing_Loads]
  [Blade_Bearing_Load_1] -> Mux1/1
  [Blade_Bearing_Load_2] -> Mux1/2
  [Blade_Bearing_Load_3] -> Mux1/3
  Mux/1 -> [Blade_Pitch]
  [Blade_Pitch_1] -> Mux/1
  [Blade_Pitch_2] -> Mux/2
  [Blade_Pitch_3] -> Mux/3

== system Pitch_System_Lib/Hydraulic/Pitch_1 ==
  Joint Sensor : mblibv1/Sensors &  Actuators/Joint Sensor  SystemSampleTime=-1  UpdateFromCAD=off  PhysicalDomain=Mechanical  PortType=blob  Muxed=off  Pose=off  Angle=on  AngleUnits=rad  ArcVelocity=off  ArcVelocityUnits=rad/s  ArcAcceleration=off  ArcAccelerationUnits=deg/s^2  CoordPosition=on  CoordPositionUnits=m  Velocity=off  VelocityUnits=m/s  Acceleration=off  AccelerationUnits=m/s^2  Quaternion=on  QuaternionDT=off  QuaternionDDT=off  QuaternionUnits=off  OutputVector=[1]  ActiveIO=off  Width=1  DialogClass=MechanicalSensorBlock  Primitive=R1  Force=off  ForceUnits=N  Torque=off  TorqueUnits=N*m  ReferenceFrame=Absolute (World)  ReactionSensedSide=Base  ReactionReferenceFrame=Absolute (World)  ReactionForce=on  ReactionForceUnits=N  ReactionMoment=on  ReactionMomentUnits=N*m
  Mux : Mux  Inputs=2
  S : PMIOPort  Tag=PMCPort  Port=1  Side=Left
  tag scope: Blade_Bearing_Load_1=global, Blade_Pitch_1=global
  wires:
  Mux/1 -> [Blade_Bearing_Load_1]
  Joint Sensor/3 -> Mux/2
  Joint Sensor/2 -> Mux/1
  Joint Sensor/1 -> [Blade_Pitch_1]
  connections:
  S/RConn1 -- Joint Sensor/LConn1

== system Pitch_System_Lib/Hydraulic/Pitch_2 ==
  Joint Sensor : mblibv1/Sensors &  Actuators/Joint Sensor  SystemSampleTime=-1  UpdateFromCAD=off  PhysicalDomain=Mechanical  PortType=blob  Muxed=off  Pose=off  Angle=on  AngleUnits=rad  ArcVelocity=off  ArcVelocityUnits=rad/s  ArcAcceleration=off  ArcAccelerationUnits=deg/s^2  CoordPosition=on  CoordPositionUnits=m  Velocity=off  VelocityUnits=m/s  Acceleration=off  AccelerationUnits=m/s^2  Quaternion=on  QuaternionDT=off  QuaternionDDT=off  QuaternionUnits=off  OutputVector=[1]  ActiveIO=off  Width=1  DialogClass=MechanicalSensorBlock  Primitive=R1  Force=off  ForceUnits=N  Torque=off  TorqueUnits=N*m  ReferenceFrame=Absolute (World)  ReactionSensedSide=Base  ReactionReferenceFrame=Absolute (World)  ReactionForce=on  ReactionForceUnits=N  ReactionMoment=on  ReactionMomentUnits=N*m
  Mux : Mux  Inputs=2
  S : PMIOPort  Tag=PMCPort  Port=1  Side=Left
  tag scope: Blade_Bearing_Load_2=global, Blade_Pitch_2=global
  wires:
  Joint Sensor/1 -> [Blade_Pitch_2]
  Joint Sensor/2 -> Mux/1
  Joint Sensor/3 -> Mux/2
  Mux/1 -> [Blade_Bearing_Load_2]
  connections:
  S/RConn1 -- Joint Sensor/LConn1

== system Pitch_System_Lib/Hydraulic/Pitch_3 ==
  Joint Sensor : mblibv1/Sensors &  Actuators/Joint Sensor  SystemSampleTime=-1  UpdateFromCAD=off  PhysicalDomain=Mechanical  PortType=blob  Muxed=off  Pose=off  Angle=on  AngleUnits=rad  ArcVelocity=off  ArcVelocityUnits=rad/s  ArcAcceleration=off  ArcAccelerationUnits=deg/s^2  CoordPosition=on  CoordPositionUnits=m  Velocity=off  VelocityUnits=m/s  Acceleration=off  AccelerationUnits=m/s^2  Quaternion=on  QuaternionDT=off  QuaternionDDT=off  QuaternionUnits=off  OutputVector=[1]  ActiveIO=off  Width=1  DialogClass=MechanicalSensorBlock  Primitive=R1  Force=off  ForceUnits=N  Torque=off  TorqueUnits=N*m  ReferenceFrame=Absolute (World)  ReactionSensedSide=Base  ReactionReferenceFrame=Absolute (World)  ReactionForce=on  ReactionForceUnits=N  ReactionMoment=on  ReactionMomentUnits=N*m
  Mux : Mux  Inputs=2
  S : PMIOPort  Tag=PMCPort  Port=1  Side=Left
  tag scope: Blade_Bearing_Load_3=global, Blade_Pitch_3=global
  wires:
  Mux/1 -> [Blade_Bearing_Load_3]
  Joint Sensor/3 -> Mux/2
  Joint Sensor/2 -> Mux/1
  Joint Sensor/1 -> [Blade_Pitch_3]
  connections:
  S/RConn1 -- Joint Sensor/LConn1
